simulink model "ChiefMaster_TTC580"  (R2022b)
settings: Solver=FixedStepAuto  StartTime=0.0  StopTime=10  FixedStep=0.01  RelTol=1e-3
values from neighbouring files (symbols this model uses):
  BattBox1_No = single(1)    [Parameters.m]
  BattBox2_No = single(2)    [Parameters.m]
  BattBox3_No = single(3)    [Parameters.m]
  CurrentLB = single(-3)    [Parameters.m]
  CurrentReductionConstant_Lvl0 = single(0.03)    [Parameters.m]
  CurrentReductionConstant_Lvl1 = single(0.05)    [Parameters.m]
  CurrentReductionConstant_Lvl2 = single(0.07)    [Parameters.m]
  CurrentReductionConstant_Lvl3 = single(0.1)    [Parameters.m]
  CurrentUB = single(3)    [Parameters.m]
  DCHV_Minus_In_Delay_ms = single(500)    [Parameters.m]
  FL_sHVC_CellBalanceVoltage_mV = single(3500)    [Parameters.m]
  FL_sInrushCurrent_dividebyzero = single(0.00001)    [Parameters.m]
  FL_u8HMI_BuzzerTimer = uint8(3)    [Parameters.m]
  IP_boActValue = true    [Parameters.m]
  IP_boDeactValue = false    [Parameters.m]
  IP_boInitValue = false    [Parameters.m]
  IP_s_LB = 18000    [Parameters.m]
  IP_s_UB = 22000    [Parameters.m]
  IP_sBatt1_ChargeCurrentMax_Factor = single(0.1)    [Parameters.m]
  IP_sBatt1_ChargeCurrentMax_LB = single(0)    [Parameters.m]
  IP_sBatt1_ChargeCurrentMax_Offset = single(0)    [Parameters.m]
  IP_sBatt1_ChargeCurrentMax_UB = single(6553.5)    [Parameters.m]
  IP_sBatt1_Current_Factor = single(0.1)    [Parameters.m]
  IP_sBatt1_Current_LB = single(-3276.8)    [Parameters.m]
  IP_sBatt1_Current_Offset = single(0)    [Parameters.m]
  IP_sBatt1_Current_UB = single(3276.8)    [Parameters.m]
  IP_sBatt1_DisChargeCurrentMax_Factor = single(0.1)    [Parameters.m]
  IP_sBatt1_DisChargeCurrentMax_LB = single(0)    [Parameters.m]
  IP_sBatt1_DisChargeCurrentMax_Offset = single(0)    [Parameters.m]
  IP_sBatt1_DisChargeCurrentMax_UB = single(6553.5)    [Parameters.m]
  IP_sBatt1_InsulationResistance_Factor = single(5)    [Parameters.m]
  IP_sBatt1_InsulationResistance_LB = single(0)    [Parameters.m]
  IP_sBatt1_InsulationResistance_Offset = single(0)    [Parameters.m]
  IP_sBatt1_InsulationResistance_UB = single(0)    [Parameters.m]
  IP_sBatt1_LiBa_IntResist_mOhm = single(25)    [Parameters.m]
  IP_sBatt1_SOC_Factor = single(1)    [Parameters.m]
  IP_sBatt1_SOC_LB = single(0)    [Parameters.m]
  IP_sBatt1_SOC_Offset = single(0)    [Parameters.m]
  IP_sBatt1_SOC_UB = single(100)    [Parameters.m]
  IP_sBatt1_SOH_Factor = single(1)    [Parameters.m]
  IP_sBatt1_SOH_LB = single(0)    [Parameters.m]
  IP_sBatt1_SOH_Offset = single(0)    [Parameters.m]
  IP_sBatt1_SOH_UB = single(100)    [Parameters.m]
  IP_sBatt1_Ubatt_Factor = single(0.1)    [Parameters.m]
  IP_sBatt1_Ubatt_LB = single(0)    [Parameters.m]
  IP_sBatt1_Ubatt_Offset = single(0)    [Parameters.m]
  IP_sBatt1_Ubatt_UB = single(6553.5)    [Parameters.m]
  IP_sBatt1_UserRi_Factor = single(1)    [Parameters.m]
  IP_sBatt1_UserRi_LB = single(0)    [Parameters.m]
  IP_sBatt1_UserRi_Offset = single(0)    [Parameters.m]
  IP_sBatt1_UserRi_UB = single(255)    [Parameters.m]
  IP_sBatt1_VoltageAtSensor_Factor = single(0.02)    [Parameters.m]
  IP_sBatt1_VoltageAtSensor_LB = single(0)    [Parameters.m]
  IP_sBatt1_VoltageAtSensor_Offset = single(0)    [Parameters.m]
  IP_sBatt1_VoltageAtSensor_UB = single(1310.7)    [Parameters.m]
  IP_sBatt2_LiBa_IntResist_mOhm = single(25)    [Parameters.m]
  IP_sBatt3_LiBa_IntResist_mOhm = single(25)    [Parameters.m]
  IP_sEM_LB = 2000    [Parameters.m]
  IP_sEM_UB = 8000    [Parameters.m]
  IP_sFB_LB = 5000    [Parameters.m]
  IP_sFB_UB = 10000    [Parameters.m]
  IP_sHVIL_LB = 12000    [Parameters.m]
  IP_sHVIL_UB = 15000    [Parameters.m]
  IP_sLoad_Voltage_Factor = single(1)    [Parameters.m]
  IP_sLoad_Voltage_LB = single(0)    [Parameters.m]
  IP_sLoad_Voltage_Offset = single(0)    [Parameters.m]
  IP_sLoad_Voltage_UB = single(65535)    [Parameters.m]
  IP_u8HVIL_Delay_ms = uint8(100)    [Parameters.m]
  IP_u8HW_IN_delay_ms = uint8(100)    [Parameters.m]
  IT_sInsulationSafeValue_kOhm = single(650)    [Parameters.m]
  IT_u8IMD_DelayTime_s = uint8(20)    [Parameters.m]
  MainHV_Minus_In_Delay = single(5)    [Parameters.m]
  MainHV_StatusDelay = single(5)    [Parameters.m]
  NotAvailable_uint16 = single(65535)    [Parameters.m]
  NotAvailable_uint8 = uint8(255)    [Parameters.m]
  OP_boHVIL_Supply = boolean(1)    [Parameters.m]
  SafeCurrentToCloseHV_A = single(5)    [Parameters.m]
  SafeVoltageToCloseHV_V = single(0.5)    [Parameters.m]
  UnexpectedBattChargingFcn_Available = boolean(1)    [Parameters.m]
  Voltage_NA_UB = uint16(65535)    [Parameters.m]
  VoltageSensorAvailableBB1 = boolean(0)    [Parameters.m]
  VoltageSensorAvailableBB2 = boolean(0)    [Parameters.m]
  VoltageSensorAvailableBB3 = boolean(0)    [Parameters.m]
libraries: simulink x184, Library_DataProcessing_v1_1 x167, Library_DataProcessing_v1 x142, libCM x28
(part 7 of 19)

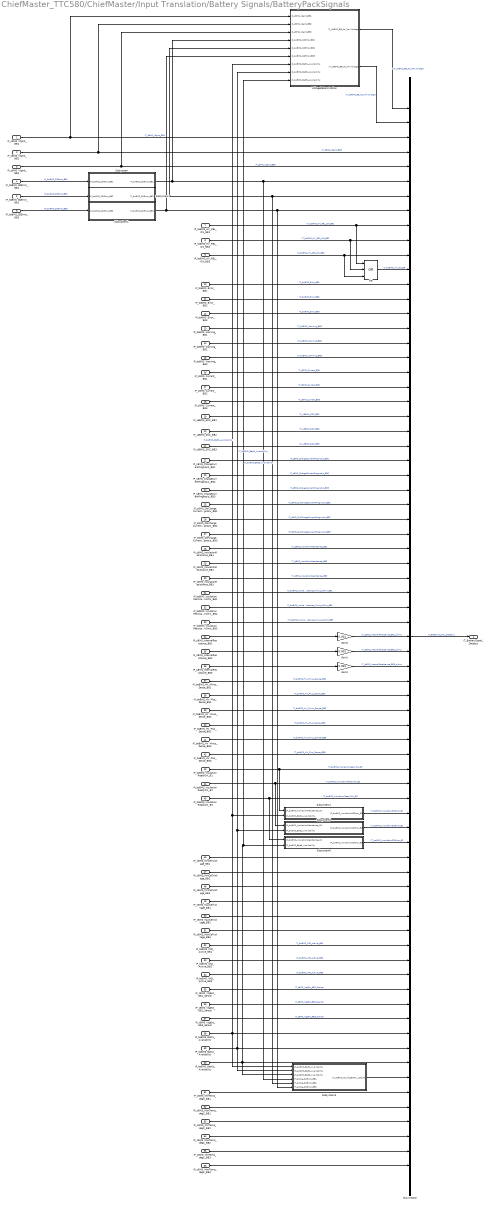
== system ChiefMaster_TTC580/ChiefMaster/Input Translation/Battery Signals/BatteryPackSignals ==
  IP_sBMS_VtgInt_BB1 : Inport
  IP_sBMS_VtgInt_BB2 : Inport  Port=2
  IP_sBMS_VtgInt_BB3 : Inport  Port=3
  IP_boBMS_SDError_BB1 : Inport  Port=4
  IP_boBMS_SDError_BB2 : Inport  Port=5
  IP_boBMS_SDError_BB3 : Inport  Port=6
  IP_boBMS_HV_REL_ON_BB1 : Inport  Port=7
  IP_boBMS_HV_REL_ON_BB2 : Inport  Port=8
  IP_boBMS_HV_REL_ON_BB3 : Inport  Port=9
  IP_boBMS_Error_BB1 : Inport  Port=10
  IP_boBMS_Error_BB2 : Inport  Port=11
  IP_boBMS_Error_BB3 : Inport  Port=12
  IP_boBMS_Warning_BB1 : Inport  Port=13
  IP_boBMS_Warning_BB2 : Inport  Port=14
  IP_boBMS_Warning_BB3 : Inport  Port=15
  IP_sBMS_Current_BB1 : Inport  Port=16
  IP_sBMS_Current_BB2 : Inport  Port=17
  IP_sBMS_Current_BB3 : Inport  Port=18
  IP_u8BMS_SOC_BB1 : Inport  Port=19
  IP_u8BMS_SOC_BB2 : Inport  Port=20
  IP_u8BMS_SOC_BB3 : Inport  Port=21
  IP_sBMS_ChargeCurrentPrognosis_BB1 : Inport  Port=22
  IP_sBMS_ChargeCurrentPrognosis_BB2 : Inport  Port=23
  IP_sBMS_ChargeCurrentPrognosis_BB3 : Inport  Port=24
  IP_sBMS_DisChargeCurrentPrognosis_BB1 : Inport  Port=25
  IP_sBMS_DisChargeCurrentPrognosis_BB2 : Inport  Port=26
  IP_sBMS_DisChargeCurrentPrognosis_BB3 : Inport  Port=27
  IP_sBMS_InsulationResistance_BB1 : Inport  Port=28
  IP_sBMS_InsulationResistance_BB2 : Inport  Port=29
  IP_sBMS_InsulationResistance_BB3 : Inport  Port=30
  IP_boBMS_InsulationResistance_Minus_kOhm_BB1 : Inport  Port=31
  IP_boBMS_InsulationResistance_Minus_kOhm_BB2 : Inport  Port=32
  IP_boBMS_InsulationResistance_Minus_kOhm_BB3 : Inport  Port=33
  IP_sBMS_InternalResistance_BB1 : Inport  Port=34
  IP_sBMS_InternalResistance_BB2 : Inport  Port=35
  IP_sBMS_InternalResistance_BB3 : Inport  Port=36
  IP_boBMS_HV_Minus_Sense_BB1 : Inport  Port=37
  IP_boBMS_HV_Plus_Sense_BB1 : Inport  Port=38
  IP_boBMS_HV_Minus_Sense_BB2 : Inport  Port=39
  IP_boBMS_HV_Plus_Sense_BB2 : Inport  Port=40
  IP_boBMS_HV_Minus_Sense_BB3 : Inport  Port=41
  IP_boBMS_HV_Plus_Sense_BB3 : Inport  Port=42
  IP_boBMS_InsulationReadyOK_B1 : Inport  Port=43
  IP_boBMS_InsulationReadyOK_B2 : Inport  Port=44
  IP_boBMS_InsulationReadyOK_B3 : Inport  Port=45
  IP_sBMS_MinCellVoltage_BB1 : Inport  Port=46
  IP_sBMS_MinCellVoltage_BB2 : Inport  Port=47
  IP_sBMS_MinCellVoltage_BB3 : Inport  Port=48
  IP_sBMS_MaxCellVoltage_BB1 : Inport  Port=49
  IP_sBMS_MaxCellVoltage_BB2 : Inport  Port=50
  IP_sBMS_MaxCellVoltage_BB3 : Inport  Port=51
  IP_boBMS_IMD_Active_BB1 : Inport  Port=52
  IP_boBMS_IMD_Active_BB2 : Inport  Port=53
  IP_boBMS_IMD_Active_BB3 : Inport  Port=54
  IP_sBMS_VtgExt_BB1_Sensor : Inport  Port=55
  IP_sBMS_VtgExt_BB2_Sensor : Inport  Port=56
  IP_sBMS_VtgExt_BB3_Sensor : Inport  Port=57
  IP_boBMS_Batt1_Availability : Inport  Port=58
  IP_boBMS_Batt2_Availability : Inport  Port=59
  IP_boBMS_Batt3_Availability : Inport  Port=60
  IP_sBMS_MinTemp_degC_BB1 : Inport  Port=61
  IP_sBMS_MaxTemp_degC_BB1 : Inport  Port=62
  IP_sBMS_MinTemp_degC_BB2 : Inport  Port=63
  IP_sBMS_MaxTemp_degC_BB2 : Inport  Port=64
  IP_sBMS_MinTemp_degC_BB3 : Inport  Port=65
  IP_sBMS_MaxTemp_degC_BB3 : Inport  Port=66
  Bus Creator : BusCreator  Inputs=73
  Gain1 : Gain  Gain=0.001  OutDataTypeStr=single
  Gain2 : Gain  Gain=0.001  OutDataTypeStr=single
  Gain3 : Gain  Gain=0.001  OutDataTypeStr=single
  OR : Logic  Operator=OR  Inputs=3  AllPortsSameDT=off  OutDataTypeStr=boolean
  Subsystem : Subsystem
  Subsystem1 : Subsystem
  Subsystem2 : Subsystem
  Subsystem3 : Subsystem
  Subsystem4 : Subsystem
  Subsystem5 : Subsystem
  Subsystem6 : Subsystem
  VoltageDetermination : Subsystem  TreatAsAtomicUnit=on
      settings: RTWFcnNameOpts=Use subsystem name  RTWFileNameOpts=Use subsystem name
  IT_BatterySignal_Databus : Outport
  wires:
  VoltageDetermination/2(IT_u8BMS_BB_No_MinVoltage) -> Bus Creator/2  "IT_u8BMS_BB_No_MinVoltage"
  IP_sBMS_VtgInt_BB3/1 -> VoltageDetermination/3(IP_sBMS_VtgInt_BB3), Bus Creator/5  "IT_sBMS_VtgInt_BB3"
  IP_sBMS_VtgInt_BB1/1 -> VoltageDetermination/1(IP_sBMS_VtgInt_BB1), Bus Creator/3  "IT_sBMS_VtgInt_BB1"
  VoltageDetermination/1(IT_u8BMS_BB_No_MaxVoltage) -> Bus Creator/1  "IT_u8BMS_BB_No_MaxVoltage"
  IP_sBMS_VtgInt_BB2/1 -> VoltageDetermination/2(IP_sBMS_VtgInt_BB2), Bus Creator/4  "IT_sBMS_VtgInt_BB2"
  IP_boBMS_HV_REL_ON_BB3/1 -> OR/3, Bus Creator/11  "IT_boBMS_HV_REL_ON_BB3"
  IP_boBMS_HV_REL_ON_BB2/1 -> OR/2, Bus Creator/10  "IT_boBMS_HV_REL_ON_BB2"
  IP_boBMS_HV_REL_ON_BB1/1 -> OR/1, Bus Creator/9  "IT_boBMS_HV_REL_ON_BB1"
  IP_boBMS_Error_BB3/1 -> Bus Creator/15  "IT_boBMS_Error_BB3"
  IP_sBMS_Current_BB3/1 -> Bus Creator/21  "IT_sBMS_Current_BB3"
  IP_u8BMS_SOC_BB3/1 -> Bus Creator/24  "IT_u8BMS_SOC_BB3"
  IP_sBMS_ChargeCurrentPrognosis_BB2/1 -> Bus Creator/26  "IT_sBMS_ChargeCurrentPrognosis_BB2"
  IP_boBMS_Warning_BB3/1 -> Bus Creator/18  "IT_boBMS_Warning_BB3"
  IP_boBMS_Error_BB2/1 -> Bus Creator/14  "IT_boBMS_Error_BB2"
  IP_boBMS_Warning_BB2/1 -> Bus Creator/17  "IT_boBMS_Warning_BB2"
  IP_boBMS_Error_BB1/1 -> Bus Creator/13  "IT_boBMS_Error_BB1"
  IP_u8BMS_SOC_BB1/1 -> Bus Creator/22  "IT_u8BMS_SOC_BB1"
  IP_sBMS_Current_BB2/1 -> Bus Creator/20  "IT_sBMS_Current_BB2"
  IP_boBMS_Warning_BB1/1 -> Bus Creator/16  "IT_boBMS_Warning_BB1"
  IP_u8BMS_SOC_BB2/1 -> Bus Creator/23  "IT_u8BMS_SOC_BB2"
  IP_sBMS_ChargeCurrentPrognosis_BB1/1 -> Bus Creator/25  "IT_sBMS_ChargeCurrentPrognosis_BB1"
  IP_sBMS_Current_BB1/1 -> Bus Creator/19  "IT_sBMS_Current_BB1"
  OR/1 -> Bus Creator/12  "IT_boBMS_HV_ON_BB"
  Bus Creator/1 -> IT_BatterySignal_Databus/1  "IT_BatterySignal_Databus"
  IP_sBMS_InsulationResistance_BB1/1 -> Bus Creator/31  "IT_sBMS_InsulationResistance_BB1"
  IP_sBMS_DisChargeCurrentPrognosis_BB3/1 -> Bus Creator/30  "IT_sBMS_DisChargeCurrentPrognosis_BB3"
  IP_sBMS_InsulationResistance_BB2/1 -> Bus Creator/32  "IT_sBMS_InsulationResistance_BB2"
  IP_boBMS_HV_Minus_Sense_BB1/1 -> Bus Creator/40  "IT_boBMS_HV_Minus_Sense_BB1"
  IP_sBMS_DisChargeCurrentPrognosis_BB2/1 -> Bus Creator/29  "IT_sBMS_DisChargeCurrentPrognosis_BB2"
  IP_sBMS_InsulationResistance_BB3/1 -> Bus Creator/33  "IT_sBMS_InsulationResistance_BB3"
  IP_boBMS_HV_Plus_Sense_BB1/1 -> Bus Creator/41  "IT_boBMS_HV_Plus_Sense_BB1"
  IP_boBMS_HV_Minus_Sense_BB2/1 -> Bus Creator/42  "IT_boBMS_HV_Minus_Sense_BB2"
  IP_sBMS_InternalResistance_BB1/1 -> Gain3/1
  IP_boBMS_HV_Plus_Sense_BB2/1 -> Bus Creator/43  "IT_boBMS_HV_Plus_Sense_BB2"
  IP_sBMS_DisChargeCurrentPrognosis_BB1/1 -> Bus Creator/28  "IT_sBMS_DisChargeCurrentPrognosis_BB1"
  IP_boBMS_HV_Minus_Sense_BB3/1 -> Bus Creator/44  "IT_boBMS_HV_Minus_Sense_BB3"
  IP_boBMS_HV_Plus_Sense_BB3/1 -> Bus Creator/45  "IT_boBMS_HV_Plus_Sense_BB3"
  IP_sBMS_ChargeCurrentPrognosis_BB3/1 -> Bus Creator/27  "IT_sBMS_ChargeCurrentPrognosis_BB3"
  IP_sBMS_InternalResistance_BB2/1 -> Gain1/1
  IP_sBMS_InternalResistance_BB3/1 -> Gain2/1
  IP_boBMS_IMD_Active_BB1/1 -> Bus Creator/58  "IT_boBMS_IMD_Active_BB1"
  IP_boBMS_IMD_Active_BB2/1 -> Bus Creator/59  "IT_boBMS_IMD_Active_BB2"
  IP_boBMS_IMD_Active_BB3/1 -> Bus Creator/60  "IT_boBMS_IMD_Active_BB3"
  IP_sBMS_VtgExt_BB1_Sensor/1 -> Bus Creator/61  "IT_sBMS_VtgExt_BB1_Sensor"
  IP_sBMS_VtgExt_BB2_Sensor/1 -> Bus Creator/62  "IT_sBMS_VtgExt_BB2_Sensor"
  IP_sBMS_VtgExt_BB3_Sensor/1 -> Bus Creator/63  "IT_sBMS_VtgExt_BB3_Sensor"
  Gain3/1 -> Bus Creator/37  "IT_sBMS_InternalResistance_BB1_ohms"
  Gain1/1 -> Bus Creator/38  "IT_sBMS_InternalResistance_BB2_ohms"
  Gain2/1 -> Bus Creator/39  "IT_sBMS_InternalResistance_BB3_ohms"
  Subsystem2/1(IT_boBMS_SDError_BB3) -> Bus Creator/8, Subsystem3/6(IT_boSig_SDError_BB3), VoltageDetermination/6(IP_boBMS_SDError_BB3)
  Subsystem1/1(IT_boBMS_SDError_BB2) -> Bus Creator/7, Subsystem3/5(IT_boSig_SDError_BB2), VoltageDetermination/5(IP_boBMS_SDError_BB2)
  IP_boBMS_Batt1_Availability/1 -> Bus Creator/64, Subsystem3/1(IP_boBMS_Batt1_Availability), Subsystem4/2(IP_boBMS_Batt1_Availability), VoltageDetermination/7(IP_boBMS_Batt1_Availability)  "IT_boBMS_Batt1_Availability"
  IP_boBMS_Batt2_Availability/1 -> Bus Creator/65, Subsystem3/2(IP_boBMS_Batt2_Availability), VoltageDetermination/8(IP_boBMS_Batt2_Availability), Subsystem5/2(IP_boBMS_Batt2_Availability)  "IT_boBMS_Batt2_Availability"
  IP_boBMS_Batt3_Availability/1 -> Bus Creator/66, Subsystem3/3(IP_boBMS_Batt3_Availability), VoltageDetermination/9(IP_boBMS_Batt3_Availability), Subsystem6/2(IP_boBMS_Batt3_Availability)  "IT_boBMS_Batt3_Availability"
  IP_boBMS_SDError_BB3/1 -> Subsystem2/1(IP_boBMS_SDError_BB3)  "IP_boBMS_SDError_BB3"
  IP_boBMS_SDError_BB2/1 -> Subsystem1/1(IP_boBMS_SDError_BB2)  "IP_boBMS_SDError_BB2"
  Subsystem/1(IT_boBMS_SDError_BB1) -> Bus Creator/6, Subsystem3/4(IT_boSig_SDError_BB1), VoltageDetermination/4(IP_boBMS_SDError_BB1)
  IP_boBMS_SDError_BB1/1 -> Subsystem/1(IP_boBMS_SDError_BB1)  "IP_boBMS_SDError_BB1"
  Subsystem3/1(IT_u8BMS_No_of_Battery_Usable) -> Bus Creator/67
  IP_boBMS_InsulationResistance_Minus_kOhm_BB1/1 -> Bus Creator/34  "IT_boBMS_InsulationResistance_Minus_kOhm_BB1"
  IP_boBMS_InsulationResistance_Minus_kOhm_BB2/1 -> Bus Creator/35  "IT_boBMS_InsulationResistance_Minus_kOhm_BB2"
  IP_boBMS_InsulationResistance_Minus_kOhm_BB3/1 -> Bus Creator/36  "IT_boBMS_InsulationResistance_Minus_kOhm_BB3"
  IP_boBMS_InsulationReadyOK_B1/1 -> Bus Creator/46, Subsystem4/1(IP_boBMS_InsulationResistance_OK)  "IT_boBMS_InsulationReadyOK_B1"
  IP_boBMS_InsulationReadyOK_B2/1 -> Bus Creator/47, Subsystem5/1(IP_boBMS_InsulationResistance_OK)  "IT_boBMS_InsulationReadyOK_B2"
  IP_boBMS_InsulationReadyOK_B3/1 -> Bus Creator/48, Subsystem6/1(IP_boBMS_InsulationResistance_OK)  "IT_boBMS_InsulationReadyOK_B3"
  Subsystem4/1(IP_boBMS_InsulationSDError_B1) -> Bus Creator/49  "IT_boBMS_InsulationSDError_B1"
  Subsystem5/1(IP_boBMS_InsulationSDError_B2) -> Bus Creator/50  "IT_boBMS_InsulationSDError_B2"
  Subsystem6/1(IP_boBMS_InsulationSDError_B3) -> Bus Creator/51  "IT_boBMS_InsulationSDError_B3"
  IP_sBMS_MinCellVoltage_BB1/1 -> Bus Creator/52
  IP_sBMS_MinCellVoltage_BB2/1 -> Bus Creator/53
  IP_sBMS_MinCellVoltage_BB3/1 -> Bus Creator/54
  IP_sBMS_MaxCellVoltage_BB1/1 -> Bus Creator/55
  IP_sBMS_MaxCellVoltage_BB2/1 -> Bus Creator/56
  IP_sBMS_MaxCellVoltage_BB3/1 -> Bus Creator/57
  IP_sBMS_MinTemp_degC_BB1/1 -> Bus Creator/68
  IP_sBMS_MaxTemp_degC_BB1/1 -> Bus Creator/69
  IP_sBMS_MinTemp_degC_BB2/1 -> Bus Creator/70
  IP_sBMS_MaxTemp_degC_BB2/1 -> Bus Creator/71
  IP_sBMS_MinTemp_degC_BB3/1 -> Bus Creator/72
  IP_sBMS_MaxTemp_degC_BB3/1 -> Bus Creator/73

== system ChiefMaster_TTC580/ChiefMaster/Input Translation/Battery Signals/Subsystem ==
  IP_Databus : Inport
  Bus Selector1 : BusSelector  OutputSignals=IP_Actia_BatBox_DataBus.IP_Actia_Batt1_Databus.IP_sActia_Batt1_Ubatt_Databus,IP_LB_BattBox_DataBus.IP_LB_BattBox1_DataBus.IP_LB_Batt1_Status02_DataBus.IP_LB_BMS_Pack_V_Cells_DataBus,IP_Actia_BatBox_DataBus.IP_Actia_Batt2_Databus.IP_sActia_Batt2_Ubatt_Databus,IP_LB_BattBox_DataBus.IP_LB_BattBox2_DataBus.IP_LB_Batt2_Status02_DataBus.IP_LB_BMS_Pack_V_Cells_DataBus,IP_Actia_BatBox_DataBus.IP_Actia_Batt3_Databus.IP_sActia_Batt3_Ubatt_Databus,IP_LB_BattBox_DataBus.IP_LB_BattBox3_DataBus.IP_LB_Batt3_Status02_DataBus.IP_LB_BMS_Pack_V_Cells_DataBus
  Subsystem : Subsystem
  Subsystem1 : Subsystem
  Subsystem2 : Subsystem
  IP_sBMS_VtgInt_BB1 : Outport
  IP_sBMS_VtgInt_BB2 : Outport  Port=2
  IP_sBMS_VtgInt_BB3 : Outport  Port=3
  wires:
  Bus Selector1/3 -> Subsystem1/1(<IP_sBatt2_Ubatt_Databus>)  "<IP_sActia_Batt2_Ubatt_Databus>"
  Bus Selector1/5 -> Subsystem2/1(<IP_sBatt3_Ubatt_Databus>)  "<IP_sActia_Batt3_Ubatt_Databus>"
  IP_Databus/1 -> Bus Selector1/1
  Bus Selector1/4 -> Subsystem1/2(<IP_LB_BMS_Pack_V_Cells_DataBus>)  "<IP_LB_BMS_Pack_V_Cells_DataBus>"
  Bus Selector1/6 -> Subsystem2/2(<IP_LB_BMS_Pack_V_Cells_DataBus>)  "<IP_LB_BMS_Pack_V_Cells_DataBus>"
  Bus Selector1/1 -> Subsystem/1(<IP_sBatt1_Ubatt_Databus>)  "<IP_sActia_Batt1_Ubatt_Databus>"
  Bus Selector1/2 -> Subsystem/2(<IP_LB_BMS_Pack_V_Cells_DataBus>)  "<IP_LB_BMS_Pack_V_Cells_DataBus>"
  Subsystem/1(IP_sBMS_VtgInt_BB1) -> IP_sBMS_VtgInt_BB1/1
  Subsystem1/1(IP_sBMS_VtgInt_BB2) -> IP_sBMS_VtgInt_BB2/1
  Subsystem2/1(IP_sBMS_VtgInt_BB3) -> IP_sBMS_VtgInt_BB3/1

== system ChiefMaster_TTC580/ChiefMaster/Input Translation/Battery Signals/Subsystem1 ==
  IP_Databus : Inport
  Bus Selector5 : BusSelector  OutputSignals=IP_Actia_BatBox_DataBus.IP_Actia_Batt1_Databus.IP_Actia_Batt1_MyStatus1_Databus.IP_boBatt1_SDERR_activ,IP_LB_BattBox_DataBus.IP_LB_BattBox1_DataBus.IP_LB_Batt1_Status01_DataBus,IP_Actia_BatBox_DataBus.IP_Actia_Batt2_Databus.IP_Actia_Batt2_MyStatus1_Databus.IP_boBatt2_SDERR_activ,IP_LB_BattBox_DataBus.IP_LB_BattBox2_DataBus.IP_LB_Batt2_Status01_DataBus,IP_Actia_BatBox_DataBus.IP_Actia_Batt3_Databus.IP_Actia_Batt3_MyStatus1_Databus.IP_boBatt3_SDERR_activ,IP_LB_BattBox_DataBus.IP_LB_BattBox3_DataBus.IP_LB_Batt3_Status01_DataBus
  Subsystem : Subsystem
  Subsystem1 : Subsystem
  Subsystem2 : Subsystem
  IP_boBMS_SDError_BB1 : Outport
  IP_boBMS_SDError_BB2 : Outport  Port=2
  IP_boBMS_SDError_BB3 : Outport  Port=3
  wires:
  IP_Databus/1 -> Bus Selector5/1
  Bus Selector5/1 -> Subsystem/1(<IP_boBatt1_SDERR_activ>)  "<IP_boBatt1_SDERR_activ>"
  Bus Selector5/2 -> Subsystem/2(<IP_LB_Batt1_Status01_DataBus>)  "<IP_LB_Batt1_Status01_DataBus>"
  Bus Selector5/3 -> Subsystem1/1(<IP_boBatt2_SDERR_activ>)  "<IP_boBatt2_SDERR_activ>"
  Bus Selector5/4 -> Subsystem1/2(<IP_LB_Batt2_Status01_DataBus>)  "<IP_LB_Batt2_Status01_DataBus>"
  Subsystem1/1(IP_boBMS_SDError_BB2) -> IP_boBMS_SDError_BB2/1
  Bus Selector5/5 -> Subsystem2/1(<IP_boBatt3_SDERR_activ>)  "<IP_boBatt3_SDERR_activ>"
  Bus Selector5/6 -> Subsystem2/2(<IP_LB_Batt2_Status01_DataBus>)  "<IP_LB_Batt3_Status01_DataBus>"
  Subsystem2/1(IP_boBMS_SDError_BB3) -> IP_boBMS_SDError_BB3/1
  Subsystem/1(IP_boBMS_SDError_BB1) -> IP_boBMS_SDError_BB1/1

== system ChiefMaster_TTC580/ChiefMaster/Input Translation/Battery Signals/Subsystem10 ==
  IP_Databus : Inport
  IMD_Req_Databus : Inport  Port=2
  Bus Selector1 : BusSelector  OutputSignals=IP_Actia_BatBox_DataBus.IP_Actia_Batt1_Databus.Batt1_MyStatus2_Databus.IP_boBatt1_IMD_active,IP_LB_BattBox_DataBus.IP_LB_BattBox1_DataBus.IP_LB_Batt1_InsulationMonitor_DataBus.IP_LB_BMS_Pack_Leak_Pos_Raw_mV_DataBus,IP_Actia_BatBox_DataBus.IP_Actia_Batt2_Databus.Batt2_MyStatus2_Databus.IP_boBatt2_IMD_active,IP_LB_BattBox_DataBus.IP_LB_BattBox2_DataBus.IP_LB_Batt2_InsulationMonitor_DataBus.IP_LB_BMS_Pack_Leak_Pos_Raw_mV_DataBus,IP_Actia_BatBox_DataBus.IP_Actia_Batt3_Databus.Batt3_MyStatus2_Databus.IP_boBatt3_IMD_active,IP_LB_BattBox_DataBus.IP_LB_BattBox3_DataBus.IP_LB_Batt3_InsulationMonitor_DataBus.IP_LB_BMS_Pack_Leak_Pos_Raw_mV_DataBus
  Subsystem1 : Subsystem
  Subsystem2 : Subsystem
  Subsystem3 : Subsystem
  Terminator : Terminator
  Terminator1 : Terminator
  Terminator2 : Terminator
  IP_boBMS_IMD_Active_BB1 : Outport
  IP_boBMS_IMD_Active_BB2 : Outport  Port=2
  IP_boBMS_IMD_Active_BB3 : Outport  Port=3
  wires:
  Subsystem3/1(IP_boBMS_IMD_Active_BB1) -> IP_boBMS_IMD_Active_BB1/1
  Bus Selector1/2 -> Terminator/1  "<IP_LB_BMS_Pack_Leak_Pos_Raw_mV_DataBus>"
  Bus Selector1/5 -> Subsystem2/1(<IP_boBMS_IMD_Active_BB3>)  "<IP_boBatt3_IMD_active>"
  Bus Selector1/3 -> Subsystem1/1(<IP_boBMS_IMD_Active_BB2>)  "<IP_boBatt2_IMD_active>"
  IP_Databus/1 -> Bus Selector1/1
  Subsystem1/1(IP_boBMS_IMD_Active_BB2) -> IP_boBMS_IMD_Active_BB2/1
  Subsystem2/1(IP_boBMS_IMD_Active_BB3) -> IP_boBMS_IMD_Active_BB3/1
  IMD_Req_Databus/1 -> Subsystem2/2(IMD_Req_Databus), Subsystem1/2(IMD_Req_Databus), Subsystem3/2("IMD_Req_Databus  ")
  Bus Selector1/4 -> Terminator1/1  "<IP_LB_BMS_Pack_Leak_Pos_Raw_mV_DataBus>"
  Bus Selector1/6 -> Terminator2/1  "<IP_LB_BMS_Pack_Leak_Pos_Raw_mV_DataBus>"
  Bus Selector1/1 -> Subsystem3/1(<IP_boBatt1_IMD_Active)  "<IP_boBatt1_IMD_active>"

== system ChiefMaster_TTC580/ChiefMaster/Input Translation/Battery Signals/Subsystem11 ==
  IP_Databus : Inport
  Bus Selector19 : BusSelector  OutputSignals=IP_Actia_BatBox_DataBus.IP_Actia_Batt1_Databus.IP_sActia_Batt1_UserRi_mOhms_DataBus,IP_Actia_BatBox_DataBus.IP_Actia_Batt2_Databus.IP_sActia_Batt2_UserRi_mOhms_DataBus,IP_Actia_BatBox_DataBus.IP_Actia_Batt3_Databus.IP_sActia_Batt3_UserRi_mOhms_DataBus
  Subsystem1 : Subsystem
  Subsystem2 : Subsystem
  Subsystem3 : Subsystem
  IP_sBMS_InternalResistance_BB1 : Outport
  IP_sBMS_InternalResistance_BB2 : Outport  Port=2
  IP_sBMS_InternalResistance_BB3 : Outport  Port=3
  wires:
  Subsystem3/1(IP_sBMS_InternalResistance_BB1) -> IP_sBMS_InternalResistance_BB1/1
  IP_Databus/1 -> Bus Selector19/1
  Bus Selector19/1 -> Subsystem3/1(<IP_sBatt1_UserRi_mOhms_DataBus>)  "<IP_sActia_Batt1_UserRi_mOhms_DataBus>"
  Bus Selector19/2 -> Subsystem1/1(<IP_sBatt2_UserRi_mOhms_DataBus>)  "<IP_sActia_Batt2_UserRi_mOhms_DataBus>"
  Bus Selector19/3 -> Subsystem2/1(<IP_sBatt3_UserRi_mOhms_DataBus>)  "<IP_sActia_Batt3_UserRi_mOhms_DataBus>"
  Subsystem1/1(IP_sBMS_InternalResistance_BB2) -> IP_sBMS_InternalResistance_BB2/1
  Subsystem2/1(IP_sBMS_InternalResistance_BB3) -> IP_sBMS_InternalResistance_BB3/1

== system ChiefMaster_TTC580/ChiefMaster/Input Translation/Battery Signals/Subsystem12 ==
  IP_Databus : Inport
  Bus Selector1 : BusSelector  OutputSignals=IP_Actia_BatBox_DataBus.IP_Actia_Batt1_Databus.IP_sActia_Batt1_InsulationResistance_kOhms_DataBus,IP_LB_BattBox_DataBus.IP_LB_BattBox1_DataBus.IP_LB_Batt1_InsulationMonitor_DataBus.IP_LB_BMS_Pack_Leak_Pos_Raw_mV_DataBus,IP_LB_BattBox_DataBus.IP_LB_BattBox1_DataBus.IP_LB_Batt1_InsulationMonitor_DataBus.IP_LB_BMS_Pack_Leak_Neg_Raw_mV_DataBus,IP_LB_BattBox_DataBus.IP_LB_BattBox1_DataBus.IP_LB_Batt1_Status02_DataBus.IP_LB_BMS_Pack_V_Cells_DataBus,IP_Actia_BatBox_DataBus.IP_Actia_Batt2_Databus.IP_sActia_Batt2_InsulationResistance_kOhms_DataBus,IP_LB_BattBox_DataBus.IP_LB_BattBox2_DataBus.IP_LB_Batt2_InsulationMonitor_DataBus.IP_LB_BMS_Pack_Leak_Pos_Raw_mV_DataBus,IP_LB_BattBox_DataBus.IP_LB_BattBox2_DataBus.IP_LB_Batt2_InsulationMonitor_DataBus.IP_LB_BMS_Pack_Leak_Neg_Raw_mV_DataBus,IP_LB_BattBox_DataBus.IP_LB_BattBox2_DataBus.IP_LB_Batt2_Status02_DataBus.IP_LB_BMS_Pack_V_Cells_DataBus,IP_Actia_BatBox_DataBus.IP_Actia_Batt3_Databus.IP_sActia_Batt3_InsulationResistance_kOhms_DataBus,IP_LB_BattBox_DataBus.IP_LB_BattBox3_DataBus.IP_LB_Batt3_InsulationMonitor_DataBus.IP_LB_BMS_Pack_Leak_Pos_Raw_mV_DataBus,IP_LB_BattBox_DataBus.IP_LB_BattBox3_DataBus.IP_LB_Batt3_InsulationMonitor_DataBus.IP_LB_BMS_Pack_Leak_Neg_Raw_mV_DataBus,IP_LB_BattBox_DataBus.IP_LB_BattBox3_DataBus.IP_LB_Batt3_Status02_DataBus.IP_LB_BMS_Pack_V_Cells_DataBus
  Subsystem1 : Subsystem
  Subsystem2 : Subsystem
  Subsystem3 : Subsystem
  IP_boBMS_InsulationResistance_kOhm_BB1 : Outport  OutDataTypeStr=single
  IP_boBMS_InsulationResistance_kOhm_BB2 : Outport  Port=2  OutDataTypeStr=single
  IP_boBMS_InsulationResistance_kOhm_BB3 : Outport  Port=3  OutDataTypeStr=single
  IP_boBMS_InsulationResistance_Minus_kOhm_BB1 : Outport  Port=4  OutDataTypeStr=single
  IP_boBMS_InsulationResistance_Minus_kOhm_BB2 : Outport  Port=5  OutDataTypeStr=single
  IP_boBMS_InsulationResistance_Minus_kOhm_BB3 : Outport  Port=6  OutDataTypeStr=single
  IP_LiBa_Insulation_OK_BB1 : Outport  Port=7
  IP_LiBa_Insulation_OK_BB2 : Outport  Port=8
  IP_LiBa_Insulation_OK_BB3 : Outport  Port=9
  wires:
  Bus Selector1/6 -> Subsystem1/2(<IP_LB_BMS_Pack_Leak_Pos_Raw_mV_DataBus>)  "<IP_LB_BMS_Pack_Leak_Pos_Raw_mV_DataBus>"
  Bus Selector1/10 -> Subsystem2/2(<IP_LB_BMS_Pack_Leak_Pos_Raw_mV_DataBus>)  "<IP_LB_BMS_Pack_Leak_Pos_Raw_mV_DataBus>"
  IP_Databus/1 -> Bus Selector1/1
  Bus Selector1/8 -> Subsystem1/4(<IP_LB_BMS_Pack_V_Cells_DataBus>)  "<IP_LB_BMS_Pack_V_Cells_DataBus>"
  Bus Selector1/12 -> Subsystem2/4(<IP_LB_BMS_Pack_V_Cells_DataBus>)  "<IP_LB_BMS_Pack_V_Cells_DataBus>"
  Bus Selector1/2 -> Subsystem3/2(<IP_LB_BMS_Pack_Leak_Pos_Raw_mV_DataBus>)  "<IP_LB_BMS_Pack_Leak_Pos_Raw_mV_DataBus>"
  Bus Selector1/4 -> Subsystem3/4(<IP_LB_BMS_Pack_V_Cells_DataBus>)  "<IP_LB_BMS_Pack_V_Cells_DataBus>"
  Bus Selector1/1 -> Subsystem3/1(<IP_sBatt1_InsulationResistance_kOhms_DataBus>)  "<IP_sActia_Batt1_InsulationResistance_kOhms_DataBus>"
  Bus Selector1/5 -> Subsystem1/1(<IP_sBatt2_InsulationResistance_kOhms_DataBus>)  "<IP_sActia_Batt2_InsulationResistance_kOhms_DataBus>"
  Subsystem2/1(IP_boBMS_InsulationResistance_kOhm_B3) -> IP_boBMS_InsulationResistance_kOhm_BB3/1
  Bus Selector1/9 -> Subsystem2/1(<IP_sBatt3_InsulationResistance_kOhms_DataBus>)  "<IP_sActia_Batt3_InsulationResistance_kOhms_DataBus>"
  Bus Selector1/3 -> Subsystem3/3(<IP_LB_BMS_Pack_Leak_Neg_Raw_mV_DataBus>)  "<IP_LB_BMS_Pack_Leak_Neg_Raw_mV_DataBus>"
  Bus Selector1/7 -> Subsystem1/3(<IP_LB_BMS_Pack_Leak_Neg_Raw_mV_DataBus>)  "<IP_LB_BMS_Pack_Leak_Neg_Raw_mV_DataBus>"
  Bus Selector1/11 -> Subsystem2/3(<IP_LB_BMS_Pack_Leak_Neg_Raw_mV_DataBus>)  "<IP_LB_BMS_Pack_Leak_Neg_Raw_mV_DataBus>"
  Subsystem2/3(IP_LiBa_Insulation_Ok_Batt3) -> IP_LiBa_Insulation_OK_BB3/1
  Subsystem2/2(IP_sLiBa_InsulationRes_Minus_BB3_kOhm) -> IP_boBMS_InsulationResistance_Minus_kOhm_BB3/1
  Subsystem3/2(IP_boBMS_InsulationResistance_Minus_kOhm_BB1) -> IP_boBMS_InsulationResistance_Minus_kOhm_BB1/1
  Subsystem3/1(IP_boBMS_InsulationResistance_kOhm_BB1) -> IP_boBMS_InsulationResistance_kOhm_BB1/1
  Subsystem3/3(IP_LiBa_Insulation_OK_BB1) -> IP_LiBa_Insulation_OK_BB1/1
  Subsystem1/1(IP_boBMS_InsulationResistance_kOhm_BB1) -> IP_boBMS_InsulationResistance_kOhm_BB2/1
  Subsystem1/3(IP_LiBa_Insulation_OK_BB1) -> IP_LiBa_Insulation_OK_BB2/1
  Subsystem1/2(IP_boBMS_InsulationResistance_Minus_kOhm_BB1) -> IP_boBMS_InsulationResistance_Minus_kOhm_BB2/1

== system ChiefMaster_TTC580/ChiefMaster/Input Translation/Battery Signals/Subsystem14 ==
  IP_Databus : Inport
  Bus Selector26 : BusSelector  OutputSignals=IP_Actia_BatBox_DataBus.IP_Actia_Batt1_Databus.IP_sActia_Batt1_MinCellVolt_mV_DataBus,IP_LB_BattBox_DataBus.IP_LB_BattBox1_DataBus.IP_LB_Batt1_CellVoltage01_DataBus.IP_LB_BMS_ACT_Cel_mV_Min_DataBus,IP_Actia_BatBox_DataBus.IP_Actia_Batt2_Databus.IP_sActia_Batt2_MinCellVolt_mV_DataBus,IP_LB_BattBox_DataBus.IP_LB_BattBox2_DataBus.IP_LB_Batt2_CellVoltage01_DataBus.IP_LB_BMS_ACT_Cel_mV_Min_DataBus,IP_Actia_BatBox_DataBus.IP_Actia_Batt3_Databus.IP_sActia_Batt3_MinCellVolt_mV_DataBus,IP_LB_BattBox_DataBus.IP_LB_BattBox3_DataBus.IP_LB_Batt3_CellVoltage01_DataBus.IP_LB_BMS_ACT_Cel_mV_Min_DataBus,IP_Actia_BatBox_DataBus.IP_Actia_Batt1_Databus.IP_sActia_Batt1_MaxCellVolt_mV_DataBus,IP_LB_BattBox_DataBus.IP_LB_BattBox1_DataBus.IP_LB_Batt1_CellVoltage01_DataBus.IP_LB_BMS_ACT_Cel_mV_Max_DataBus,IP_Actia_BatBox_DataBus.IP_Actia_Batt2_Databus.IP_sActia_Batt2_MaxCellVolt_mV_DataBus,IP_LB_BattBox_DataBus.IP_LB_BattBox2_DataBus.IP_LB_Batt2_CellVoltage01_DataBus.IP_LB_BMS_ACT_Cel_mV_Max_DataBus,IP_Actia_BatBox_DataBus.IP_Actia_Batt3_Databus.IP_sActia_Batt3_MaxCellVolt_mV_DataBus,IP_LB_BattBox_DataBus.IP_LB_BattBox3_DataBus.IP_LB_Batt3_CellVoltage01_DataBus.IP_LB_BMS_ACT_Cel_mV_Max_DataBus
  Subsystem1 : Subsystem
  Subsystem2 : Subsystem
  Subsystem3 : Subsystem
  Subsystem4 : Subsystem
  Subsystem5 : Subsystem
  Subsystem6 : Subsystem
  IP_sBMS_MinCellVoltage_BB1 : Outport
  IP_sBMS_MinCellVoltage_BB2 : Outport  Port=2
  IP_sBMS_MinCellVoltage_BB3 : Outport  Port=3
  IP_sBMS_MaxCellVoltage_BB1 : Outport  Port=4
  IP_sBMS_MaxCellVoltage_BB2 : Outport  Port=5
  IP_sBMS_MaxCellVoltage_BB3 : Outport  Port=6
  wires:
  Bus Selector26/12 -> Subsystem5/2(<IP_LB_BMS_ACT_Cel_mV_Min_DataBus>)  "<IP_LB_BMS_ACT_Cel_mV_Max_DataBus>"
  Bus Selector26/10 -> Subsystem4/2(<IP_LB_BMS_ACT_Cel_mV_Min_DataBus>)  "<IP_LB_BMS_ACT_Cel_mV_Max_DataBus>"
  Bus Selector26/8 -> Subsystem6/2(<IP_LB_BMS_ACT_Cel_mV_Min_DataBus>)  "<IP_LB_BMS_ACT_Cel_mV_Max_DataBus>"
  Bus Selector26/6 -> Subsystem2/2(<IP_LB_BMS_ACT_Cel_mV_Min_DataBus>)  "<IP_LB_BMS_ACT_Cel_mV_Min_DataBus>"
  Bus Selector26/4 -> Subsystem1/2(<IP_LB_BMS_ACT_Cel_mV_Min_DataBus>)  "<IP_LB_BMS_ACT_Cel_mV_Min_DataBus>"
  Bus Selector26/2 -> Subsystem3/2(<IP_LB_BMS_ACT_Cel_mV_Min_DataBus>)  "<IP_LB_BMS_ACT_Cel_mV_Min_DataBus>"
  IP_Databus/1 -> Bus Selector26/1
  Bus Selector26/1 -> Subsystem3/1(<IP_sActia_Batt1_MinCellVolt_mV_DataBus>)  "<IP_sActia_Batt1_MinCellVolt_mV_DataBus>"
  Bus Selector26/3 -> Subsystem1/1(<IP_sActia_Batt2_MinCellVolt_DataBus>)  "<IP_sActia_Batt2_MinCellVolt_mV_DataBus>"
  Bus Selector26/5 -> Subsystem2/1(<IP_sActia_Batt3_MinCellVolt_DataBus>)  "<IP_sActia_Batt3_MinCellVolt_mV_DataBus>"
  Bus Selector26/7 -> Subsystem6/1(<IP_sActia_Batt1_MaxCellVolt_DataBus>)  "<IP_sActia_Batt1_MaxCellVolt_mV_DataBus>"
  Bus Selector26/9 -> Subsystem4/1(<IP_sActia_Batt2_MaxCellVolt_DataBus>)  "<IP_sActia_Batt2_MaxCellVolt_mV_DataBus>"
  Bus Selector26/11 -> Subsystem5/1(<IP_sActia_Batt3_MaxCellVolt_DataBus>)  "<IP_sActia_Batt3_MaxCellVolt_mV_DataBus>"
  Subsystem3/1(IP_sBMS_MinCellVoltage_BB1) -> IP_sBMS_MinCellVoltage_BB1/1
  Subsystem1/1(IP_sBMS_MinCellVoltage_BB2) -> IP_sBMS_MinCellVoltage_BB2/1
  Subsystem2/1(IP_sBMS_MinCellVoltage_BB3) -> IP_sBMS_MinCellVoltage_BB3/1
  Subsystem6/1(IP_sBMS_MaxCellVoltage_BB1) -> IP_sBMS_MaxCellVoltage_BB1/1
  Subsystem4/1(IP_sBMS_MaxCellVoltage_BB2) -> IP_sBMS_MaxCellVoltage_BB2/1
  Subsystem5/1(IP_sBMS_MaxCellVoltage_BB3) -> IP_sBMS_MaxCellVoltage_BB3/1

== system ChiefMaster_TTC580/ChiefMaster/Input Translation/Battery Signals/Subsystem15 ==
  IP_Databus : Inport
  Bus Selector6 : BusSelector  OutputSignals=IP_Actia_BatBox_DataBus.IP_Actia_Batt1_Databus.IP_sActia_Batt1_MinTemp_degC_DataBus,IP_LB_BattBox_DataBus.IP_LB_BattBox1_DataBus.IP_LB_Batt1_CellTemperature_DataBus.IP_LB_BMS_ACT_Cel_T_Min_Value_DataBus,IP_Actia_BatBox_DataBus.IP_Actia_Batt1_Databus.IP_sActia_Batt1_MaxTemp_degC_DataBus,IP_LB_BattBox_DataBus.IP_LB_BattBox1_DataBus.IP_LB_Batt1_CellTemperature_DataBus.IP_LB_BMS_ACT_Cel_T_Max_Value_DataBus,IP_Actia_BatBox_DataBus.IP_Actia_Batt2_Databus.IP_sActia_Batt2_MinTemp_degC_DataBus,IP_LB_BattBox_DataBus.IP_LB_BattBox2_DataBus.IP_LB_Batt2_CellTemperature_DataBus.IP_LB_BMS_ACT_Cel_T_Min_Value_DataBus,IP_Actia_BatBox_DataBus.IP_Actia_Batt2_Databus.IP_sActia_Batt2_MaxTemp_degC_DataBus,IP_LB_BattBox_DataBus.IP_LB_BattBox2_DataBus.IP_LB_Batt2_CellTemperature_DataBus.IP_LB_BMS_ACT_Cel_T_Max_Value_DataBus,IP_Actia_BatBox_DataBus.IP_Actia_Batt3_Databus.IP_sActia_Batt3_MinTemp_degC_DataBus,IP_LB_BattBox_DataBus.IP_LB_BattBox3_DataBus.IP_LB_Batt3_CellTemperature_DataBus.IP_LB_BMS_ACT_Cel_T_Min_Value_DataBus,IP_Actia_BatBox_DataBus.IP_Actia_Batt3_Databus.IP_sActia_Batt3_MaxTemp_degC_DataBus,IP_LB_BattBox_DataBus.IP_LB_BattBox3_DataBus.IP_LB_Batt3_CellTemperature_DataBus.IP_LB_BMS_ACT_Cel_T_Max_Value_DataBus
  Subsystem1 : Subsystem
  Subsystem2 : Subsystem
  Subsystem3 : Subsystem
  Subsystem4 : Subsystem
  Subsystem5 : Subsystem
  Subsystem6 : Subsystem
  IP_sBMS_MinTemp_degC_BB1 : Outport
  IP_sBMS_MaxTemp_degC_BB1 : Outport  Port=2
  IP_sBMS_MinTemp_degC_BB2 : Outport  Port=3
  IP_sBMS_MaxTemp_degC_BB2 : Outport  Port=4
  IP_sBMS_MinTemp_degC_BB3 : Outport  Port=5
  IP_sBMS_MaxTemp_degC_BB3 : Outport  Port=6
  wires:
  Subsystem2/1(IP_sBMS_MinTemp_degC_BB2) -> IP_sBMS_MinTemp_degC_BB2/1
  Subsystem1/1(IP_sBMS_MaxTemp_degC_BB1) -> IP_sBMS_MaxTemp_degC_BB1/1
  IP_Databus/1 -> Bus Selector6/1
  Subsystem3/1(IP_sBMS_MinTemp_degC_BB1) -> IP_sBMS_MinTemp_degC_BB1/1
  Bus Selector6/2 -> Subsystem3/2(<IP_LB_BMS_ACT_Cel_T_Min_Value_DataBus>)  "<IP_LB_BMS_ACT_Cel_T_Min_Value_DataBus>"
  Bus Selector6/1 -> Subsystem3/1(<IP_sActia_Batt1_MinTemp_degC_DataBus>)  "<IP_sActia_Batt1_MinTemp_degC_DataBus>"
  Bus Selector6/5 -> Subsystem2/1(<IP_sActia_Batt2_MinTemp_degC_DataBus>)  "<IP_sActia_Batt2_MinTemp_degC_DataBus>"
  Bus Selector6/6 -> Subsystem2/2(<IP_LB_BMS_ACT_Cel_T_Min_Value_DataBus>)  "<IP_LB_BMS_ACT_Cel_T_Min_Value_DataBus>"
  Bus Selector6/4 -> Subsystem1/2(<IP_LB_BMS_ACT_Cel_T_Max_Value_DataBus>)  "<IP_LB_BMS_ACT_Cel_T_Max_Value_DataBus>"
  Bus Selector6/3 -> Subsystem1/1(<IP_sActia_Batt1_MaxTemp_degC_DataBus>)  "<IP_sActia_Batt1_MaxTemp_degC_DataBus>"
  Bus Selector6/7 -> Subsystem4/1(<IP_sActia_Batt2_MaxTemp_degC_DataBus>)  "<IP_sActia_Batt2_MaxTemp_degC_DataBus>"
  Bus Selector6/8 -> Subsystem4/2(<IP_LB_BMS_ACT_Cel_T_Max_Value_DataBus>)  "<IP_LB_BMS_ACT_Cel_T_Max_Value_DataBus>"
  Subsystem4/1(IP_sBMS_MaxTemp_degC_BB2) -> IP_sBMS_MaxTemp_degC_BB2/1
  Bus Selector6/9 -> Subsystem5/1(<IP_sActia_Batt3_MinTemp_degC_DataBus>)  "<IP_sActia_Batt3_MinTemp_degC_DataBus>"
  Bus Selector6/10 -> Subsystem5/2(<IP_LB_BMS_ACT_Cel_T_Min_Value_DataBus>)  "<IP_LB_BMS_ACT_Cel_T_Min_Value_DataBus>"
  Bus Selector6/11 -> Subsystem6/1(<IP_sActia_Batt3_MaxTemp_degC_DataBus>)  "<IP_sActia_Batt3_MaxTemp_degC_DataBus>"
  Bus Selector6/12 -> Subsystem6/2(<IP_LB_BMS_ACT_Cel_T_Max_Value_DataBus>)  "<IP_LB_BMS_ACT_Cel_T_Max_Value_DataBus>"
  Subsystem5/1(IP_sBMS_MinTemp_degC_BB3) -> IP_sBMS_MinTemp_degC_BB3/1
  Subsystem6/1(IP_sBMS_MaxTemp_degC_BB3) -> IP_sBMS_MaxTemp_degC_BB3/1

== system ChiefMaster_TTC580/ChiefMaster/Input Translation/Battery Signals/Subsystem2 ==
  IP_Databus : Inport
  Bus Selector5 : BusSelector  OutputSignals=IP_Actia_BatBox_DataBus.IP_Actia_Batt1_Databus.IP_Actia_Batt1_MyStatus1_Databus.IP_boBatt1_HV_REL_ON,IP_LB_BattBox_DataBus.IP_LB_BattBox1_DataBus.IP_LB_Batt1_Status01_DataBus.IP_LB_BMS_IO_state_Input_DataBus,IP_Actia_BatBox_DataBus.IP_Actia_Batt2_Databus.IP_Actia_Batt2_MyStatus1_Databus.IP_boBatt2_HV_REL_ON,IP_LB_BattBox_DataBus.IP_LB_BattBox2_DataBus.IP_LB_Batt2_Status01_DataBus.IP_LB_BMS_IO_state_Input_DataBus,IP_Actia_BatBox_DataBus.IP_Actia_Batt3_Databus.IP_Actia_Batt3_MyStatus1_Databus.IP_boBatt3_HV_REL_ON,IP_LB_BattBox_DataBus.IP_LB_BattBox3_DataBus.IP_LB_Batt3_Status01_DataBus.IP_LB_BMS_IO_state_Input_DataBus
  Subsystem : Subsystem
  Subsystem1 : Subsystem
  Subsystem2 : Subsystem
  IP_boBMS_HV_REL_ON_BB1 : Outport
  IP_boBMS_HV_REL_ON_BB2 : Outport  Port=2
  IP_boBMS_HV_REL_ON_BB3 : Outport  Port=3
  wires:
  Subsystem/1(IP_boBMS_HV_REL_ON_BB1) -> IP_boBMS_HV_REL_ON_BB1/1
  Bus Selector5/6 -> Subsystem2/2(IP_LB_BMS_IO_state_Input_DataBus)  "<IP_LB_BMS_IO_state_Input_DataBus>"
  Bus Selector5/5 -> Subsystem2/1(IP_boBatt3_HV_REL_ON)  "<IP_boBatt3_HV_REL_ON>"
  Bus Selector5/4 -> Subsystem1/2(IP_LB_BMS_IO_state_Input_DataBus)  "<IP_LB_BMS_IO_state_Input_DataBus>"
  Bus Selector5/3 -> Subsystem1/1(IP_boBatt2_HV_REL_ON)  "<IP_boBatt2_HV_REL_ON>"
  IP_Databus/1 -> Bus Selector5/1
  Bus Selector5/1 -> Subsystem/1(IP_boBatt1_HV_REL_ON)  "<IP_boBatt1_HV_REL_ON>"
  Bus Selector5/2 -> Subsystem/2(IP_LB_BMS_IO_state_Input_DataBus)  "<IP_LB_BMS_IO_state_Input_DataBus>"
  Subsystem1/1(IP_boBMS_HV_REL_ON_BB2) -> IP_boBMS_HV_REL_ON_BB2/1
  Subsystem2/1(IP_boBMS_HV_REL_ON_BB3) -> IP_boBMS_HV_REL_ON_BB3/1

== system ChiefMaster_TTC580/ChiefMaster/Input Translation/Battery Signals/Subsystem3 ==
  IP_Databus : Inport
  Bus Selector6 : BusSelector  OutputSignals=IP_Actia_BatBox_DataBus.IP_Actia_Batt1_Databus.IP_sActia_Batt1_SOC_percent_DataBus,IP_LB_BattBox_DataBus.IP_LB_BattBox1_DataBus.IP_LB_Batt1_Status02_DataBus.IP_LB_BMS_Pack_Q_SOC_Internal_DataBus,IP_Actia_BatBox_DataBus.IP_Actia_Batt2_Databus.IP_sActia_Batt2_SOC_percent_DataBus,IP_LB_BattBox_DataBus.IP_LB_BattBox2_DataBus.IP_LB_Batt2_Status02_DataBus.IP_LB_BMS_Pack_Q_SOC_Internal_DataBus,IP_Actia_BatBox_DataBus.IP_Actia_Batt3_Databus.IP_sActia_Batt3_SOC_percent_DataBus,IP_LB_BattBox_DataBus.IP_LB_BattBox3_DataBus.IP_LB_Batt3_Status02_DataBus.IP_LB_BMS_Pack_Q_SOC_Internal_DataBus
  Data Type Conversion : DataTypeConversion  OutDataTypeStr=uint8  SaturateOnIntegerOverflow=off  RndMeth=Floor
  Data Type Conversion1 : DataTypeConversion  OutDataTypeStr=uint8  SaturateOnIntegerOverflow=off  RndMeth=Floor
  Data Type Conversion2 : DataTypeConversion  OutDataTypeStr=uint8  SaturateOnIntegerOverflow=off  RndMeth=Floor
  Subsystem : Subsystem
  Subsystem1 : Subsystem
  Subsystem2 : Subsystem
  IP_sBMS_SOC_BB1 : Outport
  IP_sBMS_SOC_BB2 : Outport  Port=2
  IP_sBMS_SOC_BB3 : Outport  Port=3
  wires:
  Bus Selector6/6 -> Subsystem2/2(<IP_LB_BMS_Pack_Q_SOC_Internal_DataBus>)  "<IP_LB_BMS_Pack_Q_SOC_Internal_DataBus>"
  Bus Selector6/4 -> Subsystem1/2(<IP_LB_BMS_Pack_Q_SOC_Internal_DataBus>)  "<IP_LB_BMS_Pack_Q_SOC_Internal_DataBus>"
  IP_Databus/1 -> Bus Selector6/1
  Bus Selector6/3 -> Subsystem1/1(<IP_sBatt2_SOC_percent_DataBus>)  "<IP_sActia_Batt2_SOC_percent_DataBus>"
  Bus Selector6/5 -> Subsystem2/1(<IP_sBatt3_SOC_percent_DataBus>)  "<IP_sActia_Batt3_SOC_percent_DataBus>"
  Bus Selector6/1 -> Subsystem/1(<IP_sBatt1_SOC_percent_DataBus>)  "<IP_sActia_Batt1_SOC_percent_DataBus>"
  Bus Selector6/2 -> Subsystem/2(<IP_LB_BMS_Pack_Q_SOC_Internal_DataBus>)  "<IP_LB_BMS_Pack_Q_SOC_Internal_DataBus>"
  Subsystem/1(IP_sBMS_SOC_BB1) -> Data Type Conversion/1
  Subsystem1/1(IP_sBMS_SOC_BB2) -> Data Type Conversion1/1
  Subsystem2/1(IP_sBMS_SOC_BB3) -> Data Type Conversion2/1
  Data Type Conversion/1 -> IP_sBMS_SOC_BB1/1
  Data Type Conversion1/1 -> IP_sBMS_SOC_BB2/1
  Data Type Conversion2/1 -> IP_sBMS_SOC_BB3/1

== system ChiefMaster_TTC580/ChiefMaster/Input Translation/Battery Signals/Subsystem4 ==
  IP_DataBus : Inport
  Bus Selector6 : BusSelector  OutputSignals=IP_Actia_BatBox_DataBus.IP_Actia_Batt1_Databus.IP_sActia_Batt1_DisChargeCurrentMax_A_Databus,IP_LB_BattBox_DataBus.IP_LB_BattBox1_DataBus.IP_LB_Batt1_Status01_DataBus.IP_LB_BMS_DYN_Lim_Current_OUT_A_DataBus,IP_Actia_BatBox_DataBus.IP_Actia_Batt2_Databus.IP_sActia_Batt2_DisChargeCurrentMax_A_Databus,IP_LB_BattBox_DataBus.IP_LB_BattBox2_DataBus.IP_LB_Batt2_Status01_DataBus.IP_LB_BMS_DYN_Lim_Current_OUT_A_DataBus,IP_Actia_BatBox_DataBus.IP_Actia_Batt3_Databus.IP_sActia_Batt3_DisChargeCurrentMax_A_Databus,IP_LB_BattBox_DataBus.IP_LB_BattBox3_DataBus.IP_LB_Batt3_Status01_DataBus.IP_LB_BMS_DYN_Lim_Current_OUT_A_DataBus
  Subsystem : Subsystem
  Subsystem1 : Subsystem
  Subsystem2 : Subsystem
  IP_sBMS_DisChargeCurrentPrognosis_BB1 : Outport
  IP_sBMS_DisChargeCurrentPrognosis_BB2 : Outport  Port=2
  IP_sBMS_DisChargeCurrentPrognosis_BB3 : Outport  Port=3
  wires:
  IP_DataBus/1 -> Bus Selector6/1
  Subsystem/1(IP_sBMS_DisChargeCurrentPrognosis_BB1) -> IP_sBMS_DisChargeCurrentPrognosis_BB1/1
  Subsystem1/1(IP_sBMS_DisChargeCurrentPrognosis_BB2) -> IP_sBMS_DisChargeCurrentPrognosis_BB2/1
  Subsystem2/1(IP_sBMS_DisChargeCurrentPrognosis_BB2) -> IP_sBMS_DisChargeCurrentPrognosis_BB3/1
  Bus Selector6/1 -> Subsystem/1(<IP_sBatt1_DisChargeCurrentMax_A_Databus>)  "<IP_sActia_Batt1_DisChargeCurrentMax_A_Databus>"
  Bus Selector6/2 -> Subsystem/2(<IP_LB_BMS_DYN_Lim_Current_OUT_A_DataBus>)  "<IP_LB_BMS_DYN_Lim_Current_OUT_A_DataBus>"
  Bus Selector6/3 -> Subsystem1/1(<IP_sBatt2_DisChargeCurrentMax_A_Databus>)  "<IP_sActia_Batt2_DisChargeCurrentMax_A_Databus>"
  Bus Selector6/4 -> Subsystem1/2(<IP_LB_BMS_DYN_Lim_Current_OUT_A_DataBus>)  "<IP_LB_BMS_DYN_Lim_Current_OUT_A_DataBus>"
  Bus Selector6/5 -> Subsystem2/1(<IP_sBatt3_DisChargeCurrentMax_A_Databus>)  "<IP_sActia_Batt3_DisChargeCurrentMax_A_Databus>"
  Bus Selector6/6 -> Subsystem2/2(<IP_LB_BMS_DYN_Lim_Current_OUT_A_DataBus>)  "<IP_LB_BMS_DYN_Lim_Current_OUT_A_DataBus>"

== system ChiefMaster_TTC580/ChiefMaster/Input Translation/Battery Signals/Subsystem5 ==
  IP_DataBus : Inport
  Bus Selector6 : BusSelector  OutputSignals=IP_Actia_BatBox_DataBus.IP_Actia_Batt1_Databus.IP_sActia_Batt1_ChargeCurrentMax_A_Databus,IP_LB_BattBox_DataBus.IP_LB_BattBox1_DataBus.IP_LB_Batt1_Status03_DataBus.IP_LB_BMS_REQ_Charger_Current_A_DataBus,IP_LB_BattBox_DataBus.IP_LB_BattBox1_DataBus.IP_LB_Batt1_Status01_DataBus.IP_LB_BMS_DYN_Lim_Current_IN_A_DataBus,IP_Actia_BatBox_DataBus.IP_Actia_Batt2_Databus.IP_sActia_Batt2_ChargeCurrentMax_A_Databus,IP_LB_BattBox_DataBus.IP_LB_BattBox2_DataBus.IP_LB_Batt2_Status03_DataBus.IP_LB_BMS_REQ_Charger_Current_A_DataBus,IP_LB_BattBox_DataBus.IP_LB_BattBox2_DataBus.IP_LB_Batt2_Status01_DataBus.IP_LB_BMS_DYN_Lim_Current_IN_A_DataBus,IP_Actia_BatBox_DataBus.IP_Actia_Batt3_Databus.IP_sActia_Batt3_ChargeCurrentMax_A_Databus,IP_LB_BattBox_DataBus.IP_LB_BattBox3_DataBus.IP_LB_Batt3_Status03_DataBus.IP_LB_BMS_REQ_Charger_Current_A_DataBus,IP_LB_BattBox_DataBus.IP_LB_BattBox3_DataBus.IP_LB_Batt3_Status01_DataBus.IP_LB_BMS_DYN_Lim_Current_IN_A_DataBus
  Subsystem : Subsystem
  Subsystem1 : Subsystem
  Subsystem2 : Subsystem
  IP_sBMS_ChargeCurrentPrognosis_BB1 : Outport
  IP_sBMS_ChargeCurrentPrognosis_BB2 : Outport  Port=2
  IP_sBMS_ChargeCurrentPrognosis_BB3 : Outport  Port=3
  wires:
  Subsystem2/1(IP_sBMS_ChargeCurrentPrognosis_BB2) -> IP_sBMS_ChargeCurrentPrognosis_BB3/1
  Subsystem1/1(IP_sBMS_ChargeCurrentPrognosis_BB2) -> IP_sBMS_ChargeCurrentPrognosis_BB2/1
  Subsystem/1(IP_sBMS_ChargeCurrentPrognosis_BB1) -> IP_sBMS_ChargeCurrentPrognosis_BB1/1
  Bus Selector6/3 -> Subsystem/3(<IP_LB_BMS_DYN_Lim_Current_IN_A_DataBus>)  "<IP_LB_BMS_DYN_Lim_Current_IN_A_DataBus>"
  Bus Selector6/2 -> Subsystem/2(<IP_LB_BMS_REQ_Charger_Current_A_DataBus>)  "<IP_LB_BMS_REQ_Charger_Current_A_DataBus>"
  Bus Selector6/1 -> Subsystem/1(<IP_sBatt1_ChargeCurrentMax_A_Databus>)  "<IP_sActia_Batt1_ChargeCurrentMax_A_Databus>"
  Bus Selector6/4 -> Subsystem1/1(<IP_sBatt2_ChargeCurrentMax_A_Databus>)  "<IP_sActia_Batt2_ChargeCurrentMax_A_Databus>"
  Bus Selector6/5 -> Subsystem1/2(<IP_LB_BMS_REQ_Charger_Current_A_DataBus>)  "<IP_LB_BMS_REQ_Charger_Current_A_DataBus>"
  Bus Selector6/6 -> Subsystem1/3(<IP_LB_BMS_DYN_Lim_Current_IN_A_DataBus>)  "<IP_LB_BMS_DYN_Lim_Current_IN_A_DataBus>"
  Bus Selector6/7 -> Subsystem2/1(<IP_sBatt3_ChargeCurrentMax_A_Databus>)  "<IP_sActia_Batt3_ChargeCurrentMax_A_Databus>"
  Bus Selector6/9 -> Subsystem2/3(<IP_LB_BMS_DYN_Lim_Current_IN_A_DataBus>)  "<IP_LB_BMS_DYN_Lim_Current_IN_A_DataBus>"
  IP_DataBus/1 -> Bus Selector6/1
  Bus Selector6/8 -> Subsystem2/2(<IP_LB_BMS_REQ_Charger_Current_A_DataBus>)  "<IP_LB_BMS_REQ_Charger_Current_A_DataBus>"

== system ChiefMaster_TTC580/ChiefMaster/Input Translation/Battery Signals/Subsystem6 ==
  IP_Databus : Inport
  Bus Selector6 : BusSelector  OutputSignals=IP_Actia_BatBox_DataBus.IP_Actia_Batt1_Databus.IP_sActia_Batt1_Current_A_DataBus,IP_LB_BattBox_DataBus.IP_LB_BattBox1_DataBus.IP_LB_Batt1_Status02_DataBus.IP_LB_BMS_Pack_Current_Master_mA_DataBus,IP_Actia_BatBox_DataBus.IP_Actia_Batt2_Databus.IP_sActia_Batt2_Current_A_DataBus,IP_LB_BattBox_DataBus.IP_LB_BattBox2_DataBus.IP_LB_Batt2_Status02_DataBus.IP_LB_BMS_Pack_Current_Master_mA_DataBus,IP_Actia_BatBox_DataBus.IP_Actia_Batt3_Databus.IP_sActia_Batt3_Current_A_DataBus,IP_LB_BattBox_DataBus.IP_LB_BattBox3_DataBus.IP_LB_Batt3_Status02_DataBus.IP_LB_BMS_Pack_Current_Master_mA_DataBus
  Subsystem3 : Subsystem
  Subsystem4 : Subsystem
  Subsystem5 : Subsystem
  IP_sBMS_Current_BB1 : Outport
  IP_sBMS_Current_BB2 : Outport  Port=2
  IP_sBMS_Current_BB3 : Outport  Port=3
  wires:
  Bus Selector6/3 -> Subsystem4/1(<IP_sBatt2_Current_A_DataBus>)  "<IP_sActia_Batt2_Current_A_DataBus>"
  Bus Selector6/4 -> Subsystem4/2(<IP_LB_BMS_Pack_Current_Master_mA_DataBus>)  "<IP_LB_BMS_Pack_Current_Master_mA_DataBus>"
  Bus Selector6/6 -> Subsystem5/2(<IP_LB_BMS_Pack_Current_Master_mA_DataBus>)  "<IP_LB_BMS_Pack_Current_Master_mA_DataBus>"
  Bus Selector6/5 -> Subsystem5/1(<IP_sBatt3_Current_A_DataBus>)  "<IP_sActia_Batt3_Current_A_DataBus>"
  Bus Selector6/1 -> Subsystem3/1(<IP_sBatt1_Current_A_DataBus>)  "<IP_sActia_Batt1_Current_A_DataBus>"
  Bus Selector6/2 -> Subsystem3/2(<IP_LB_BMS_Pack_Current_Master_mA_DataBus>)  "<IP_LB_BMS_Pack_Current_Master_mA_DataBus>"
  Subsystem3/1(IP_sBMS_Current_BB1) -> IP_sBMS_Current_BB1/1
  IP_Databus/1 -> Bus Selector6/1
  Subsystem4/1(IP_sBMS_Current_BB2) -> IP_sBMS_Current_BB2/1
  Subsystem5/1(IP_sBMS_Current_BB3) -> IP_sBMS_Current_BB3/1

== system ChiefMaster_TTC580/ChiefMaster/Input Translation/Battery Signals/Subsystem7 ==
  IP_Databus : Inport
  IMD_Req_Databus : Inport  Port=2
  Bus Selector1 : BusSelector  OutputSignals=IP_Actia_BatBox_DataBus.IP_Actia_Batt1_Databus.IP_Actia_Batt1_MyStatus1_Databus.IP_boBatt1_Insulation_ready_and_OK,IP_HW_Input_DataBus.IP_boHW_IMD_FB_BB1,IP_Actia_BatBox_DataBus.IP_Actia_Batt2_Databus.IP_Actia_Batt2_MyStatus1_Databus.IP_boBatt2_Insulation_ready_and_OK,IP_HW_Input_DataBus.IP_boHW_IMD_FB_BB2,IP_Actia_BatBox_DataBus.IP_Actia_Batt3_Databus.IP_Actia_Batt3_MyStatus1_Databus.IP_boBatt3_Insulation_ready_and_OK,IP_HW_Input_DataBus.IP_boHW_IMD_FB_BB3
  Subsystem1 : Subsystem
  Subsystem2 : Subsystem
  Subsystem3 : Subsystem
  IP_boBMS_InsulationReadyOK_B1 : Outport
  IP_boBMS_InsulationReadyOK_B2 : Outport  Port=2
  IP_boBMS_InsulationReadyOK_B3 : Outport  Port=3
  wires:
  IP_Databus/1 -> Bus Selector1/1
  Bus Selector1/3 -> Subsystem1/1(<IP_boBatt2_Insulation_ready_and_OK>)  "<IP_boBatt2_Insulation_ready_and_OK>"
  Bus Selector1/5 -> Subsystem2/1(<IP_boBatt3_Insulation_ready_and_OK>)  "<IP_boBatt3_Insulation_ready_and_OK>"
  Bus Selector1/1 -> Subsystem3/1(<IP_boBatt1_Insulation_ready_and_OK>)  "<IP_boBatt1_Insulation_ready_and_OK>"
  Subsystem3/1(IP_boBMS_InsulationReadyOK_B1) -> IP_boBMS_InsulationReadyOK_B1/1
  Subsystem1/1(IP_boBMS_InsulationReadyOK_B2) -> IP_boBMS_InsulationReadyOK_B2/1
  Subsystem2/1(IP_boBMS_InsulationReadyOK_B3) -> IP_boBMS_InsulationReadyOK_B3/1
  Bus Selector1/2 -> Subsystem3/2(IP_LiBa_Insulation_OK_BB1)  "<IP_boHW_IMD_FB_BB1>"
  Bus Selector1/4 -> Subsystem1/2(IP_LiBa_Insulation_OK_BB2)  "<IP_boHW_IMD_FB_BB2>"
  Bus Selector1/6 -> Subsystem2/2(IP_LiBa_Insulation_OK_BB3)  "<IP_boHW_IMD_FB_BB3>"
  IMD_Req_Databus/1 -> Subsystem2/3(IMD_Req_Databus), Subsystem1/3(IMD_Req_Databus), Subsystem3/3(IMD_Req_Databus)

== system ChiefMaster_TTC580/ChiefMaster/Input Translation/Battery Signals/Subsystem8 ==
  IP_Databus : Inport
  Bus Selector26 : BusSelector  OutputSignals=IP_Actia_BatBox_DataBus.IP_Actia_Batt3_Databus.IP_sActia_Batt3_Availability,IP_LB_BattBox_DataBus.IP_LB_BattBox1_DataBus.IP_boLiBa_Batt1_Availability,IP_Actia_BatBox_DataBus.IP_Actia_Batt2_Databus.IP_sActia_Batt2_Availability,IP_LB_BattBox_DataBus.IP_LB_BattBox2_DataBus.IP_boLiBa_Batt2_Availability,IP_Actia_BatBox_DataBus.IP_Actia_Batt3_Databus.IP_sActia_Batt3_Availability,IP_LB_BattBox_DataBus.IP_LB_BattBox3_DataBus.IP_boLiBa_Batt3_Availability
  Subsystem : Subsystem
  Subsystem1 : Subsystem
  Subsystem2 : Subsystem
  IP_boBMS_Batt1_Availability : Outport
  IP_boBMS_Batt2_Availability : Outport  Port=2
  IP_boBMS_Batt3_Availability : Outport  Port=3
  wires:
  Subsystem/1(IP_boBMS_Batt1_Availability) -> IP_boBMS_Batt1_Availability/1
  IP_Databus/1 -> Bus Selector26/1
  Bus Selector26/1 -> Subsystem/1(<IP_sBatt1_Availability>)  "<IP_sActia_Batt3_Availability>"
  Bus Selector26/2 -> Subsystem/2(<IP_sLiBa_Batt1_Availability>)  "<IP_boLiBa_Batt1_Availability>"
  Bus Selector26/4 -> Subsystem1/2(<IP_sLiBa_Batt2_Availability>)  "<IP_boLiBa_Batt2_Availability>"
  Bus Selector26/3 -> Subsystem1/1(<IP_sBatt2_Availability>)  "<IP_sActia_Batt2_Availability>"
  Subsystem1/1(IP_boBMS_Batt2_Availability) -> IP_boBMS_Batt2_Availability/1
  Subsystem2/1(IP_boBMS_Batt3_Availability) -> IP_boBMS_Batt3_Availability/1
  Bus Selector26/5 -> Subsystem2/1(<IP_sBatt3_Availability>)  "<IP_sActia_Batt3_Availability>"
  Bus Selector26/6 -> Subsystem2/2(<IP_sLiBa_Batt3_Availability>)  "<IP_boLiBa_Batt3_Availability>"
